simulink model "Nmpc_pathctl_casadi"  (R2022b)
(part 8 of 11)

1961.70000000000,0;1961.80000000000,0;1961.90000000000,0;1962,0;1962.10000000000,0;1962.20000000000,0;1962.30000000000,0;1962.40000000000,0;1962.50000000000,0;1962.60000000000,0;1962.70000000000,0;1962.80000000000,0;1962.90000000000,0;1963,0;1963.10000000000,0;1963.20000000000,0;1963.30000000000,0;1963.40000000000,0;1963.50000000000,0;1963.60000000000,0;1963.70000000000,0;1963.80000000000,0;1963.90000000000,0;1964,0;1964.10000000000,0;1964.20000000000,0;1964.30000000000,0;1964.40000000000,0;1964.50000000000,0;1964.60000000000,0;1964.70000000000,0;1964.80000000000,0;1964.90000000000,0;1965,0;1965.10000000000,0;1965.20000000000,0;1965.30000000000,0;1965.40000000000,0;1965.50000000000,0;1965.60000000000,0;1965.70000000000,0;1965.80000000000,0;1965.90000000000,0;1966,0;1966.10000000000,0;1966.20000000000,0;1966.30000000000,0;1966.40000000000,0;1966.50000000000,0;1966.60000000000,0;1966.70000000000,0;1966.80000000000,0;1966.90000000000,0;1967,0;1967.10000000000,0;1967.20000000000,0;1967.30000000000,0;1967.40000000000,0;1967.50000000000,0;1967.60000000000,0;1967.70000000000,0;1967.80000000000,0;1967.90000000000,0;1968,0;1968.10000000000,0;1968.20000000000,0;1968.30000000000,0;1968.40000000000,0;1968.50000000000,0;1968.60000000000,0;1968.70000000000,0;1968.80000000000,0;1968.90000000000,0;1969,0;1969.10000000000,0;1969.20000000000,0;1969.30000000000,0;1969.40000000000,0;1969.50000000000,0;1969.60000000000,0;1969.70000000000,0;1969.80000000000,0;1969.90000000000,0;1970,0;1970.10000000000,0;1970.20000000000,0;1970.30000000000,0;1970.40000000000,0;1970.50000000000,0;1970.60000000000,0;1970.70000000000,0;1970.80000000000,0;1970.90000000000,0;1971,0;1971.10000000000,0;1971.20000000000,0;1971.30000000000,0;1971.40000000000,0;1971.50000000000,0;1971.60000000000,0;1971.70000000000,0;1971.80000000000,0;1971.90000000000,0;1972,0;1972.10000000000,0;1972.20000000000,0;1972.30000000000,0;1972.40000000000,0;1972.50000000000,0;1972.60000000000,0;1972.70000000000,0;1972.80000000000,0;1972.90000000000,0;1973,0;1973.10000000000,0;1973.20000000000,0;1973.30000000000,0;1973.40000000000,0;1973.50000000000,0;1973.60000000000,0;1973.70000000000,0;1973.80000000000,0;1973.90000000000,0;1974,0;1974.10000000000,0;1974.20000000000,0;1974.30000000000,0;1974.40000000000,0;1974.50000000000,0;1974.60000000000,0;1974.70000000000,0;1974.80000000000,0;1974.90000000000,0;1975,0;1975.10000000000,0;1975.20000000000,0;1975.30000000000,0;1975.40000000000,0;1975.50000000000,0;1975.60000000000,0;1975.70000000000,0;1975.80000000000,0;1975.90000000000,0;1976,0;1976.10000000000,0;1976.20000000000,0;1976.30000000000,0;1976.40000000000,0;1976.50000000000,0;1976.60000000000,0;1976.70000000000,0;1976.80000000000,0;1976.90000000000,0;1977,0;1977.10000000000,0;1977.20000000000,0;1977.30000000000,0;1977.40000000000,0;1977.50000000000,0;1977.60000000000,0;1977.70000000000,0;1977.80000000000,0;1977.90000000000,0;1978,0;1978.10000000000,0;1978.20000000000,0;1978.30000000000,0;1978.40000000000,0;1978.50000000000,0;1978.60000000000,0;1978.70000000000,0;1978.80000000000,0;1978.90000000000,0;1979,0;1979.10000000000,0;1979.20000000000,0;1979.30000000000,0;1979.40000000000,0;1979.50000000000,0;1979.60000000000,0;1979.70000000000,0;1979.80000000000,0;1979.90000000000,0;1980,0;1980.10000000000,0;1980.20000000000,0;1980.30000000000,0;1980.40000000000,0;1980.50000000000,0;1980.60000000000,0;1980.70000000000,0;1980.80000000000,0;1980.90000000000,0;1981,0;1981.10000000000,0;1981.20000000000,0;1981.30000000000,0;1981.40000000000,0;1981.50000000000,0;1981.60000000000,0;1981.70000000000,0;1981.80000000000,0;1981.90000000000,0;1982,0;1982.10000000000,0;1982.20000000000,0;1982.30000000000,0;1982.40000000000,0;1982.50000000000,0;1982.60000000000,0;1982.70000000000,0;1982.80000000000,0;1982.90000000000,0;1983,0;1983.10000000000,0;1983.20000000000,0;1983.30000000000,0;1983.40000000000,0;1983.50000000000,0;1983.60000000000,0;1983.70000000000,0;1983.80000000000,0;1983.90000000000,0;1984,0;1984.10000000000,0;1984.20000000000,0;1984.30000000000,0;1984.40000000000,0;1984.50000000000,0;1984.60000000000,0;1984.70000000000,0;1984.80000000000,0;1984.90000000000,0;1985,0;1985.10000000000,0;1985.20000000000,0;1985.30000000000,0;1985.40000000000,0;1985.50000000000,0;1985.60000000000,0;1985.70000000000,0;1985.80000000000,0;1985.90000000000,0;1986,0;1986.10000000000,0;1986.20000000000,0;1986.30000000000,0;1986.40000000000,0;1986.50000000000,0;1986.60000000000,0;1986.70000000000,0;1986.80000000000,0;1986.90000000000,0;1987,0;1987.10000000000,0;1987.20000000000,0;1987.30000000000,0;1987.40000000000,0;1987.50000000000,0;1987.60000000000,0;1987.70000000000,0;1987.80000000000,0;1987.90000000000,0;1988,0;1988.10000000000,0;1988.20000000000,0;1988.30000000000,0;1988.40000000000,0;1988.50000000000,0;1988.60000000000,0;1988.70000000000,0;1988.80000000000,0;1988.90000000000,0;1989,0;1989.10000000000,0;1989.20000000000,0;1989.30000000000,0;1989.40000000000,0;1989.50000000000,0;1989.60000000000,0;1989.70000000000,0;1989.80000000000,0;1989.90000000000,0;1990,0;1990.10000000000,0;1990.20000000000,0;1990.30000000000,0;1990.40000000000,0;1990.50000000000,0;1990.60000000000,0;1990.70000000000,0;1990.80000000000,0;1990.90000000000,0;1991,0;1991.10000000000,0;1991.20000000000,0;1991.30000000000,0;1991.40000000000,0;1991.50000000000,0;1991.60000000000,0;1991.70000000000,0;1991.80000000000,0;1991.90000000000,0;1992,0;1992.10000000000,0;1992.20000000000,0;1992.30000000000,0;1992.40000000000,0;1992.50000000000,0;1992.60000000000,0;1992.70000000000,0;1992.80000000000,0;1992.90000000000,0;1993,0;1993.10000000000,0;1993.20000000000,0;1993.30000000000,0;1993.40000000000,0;1993.50000000000,0;1993.60000000000,0;1993.70000000000,0;1993.80000000000,0;1993.90000000000,0;1994,0;1994.10000000000,0;1994.20000000000,0;1994.30000000000,0;1994.40000000000,0;1994.50000000000,0;1994.60000000000,0;1994.70000000000,0;1994.80000000000,0;1994.90000000000,0;1995,0;1995.10000000000,0;1995.20000000000,0;1995.30000000000,0;1995.40000000000,0;1995.50000000000,0;1995.60000000000,0;1995.70000000000,0;1995.80000000000,0;1995.90000000000,0;1996,0;1996.10000000000,0;1996.20000000000,0;1996.30000000000,0;1996.40000000000,0;1996.50000000000,0;1996.60000000000,0;1996.70000000000,0;1996.80000000000,0;1996.90000000000,0;1997,0;1997.10000000000,0;1997.20000000000,0;1997.30000000000,0;1997.40000000000,0;1997.50000000000,0;1997.60000000000,0;1997.70000000000,0;1997.80000000000,0;1997.90000000000,0;1998,0;1998.10000000000,0;1998.20000000000,0;1998.30000000000,0;1998.40000000000,0;1998.50000000000,0;1998.60000000000,0;1998.70000000000,0;1998.80000000000,0;1998.90000000000,0;1999,0;1999.10000000000,0;1999.20000000000,0;1999.30000000000,0;1999.40000000000,0;1999.50000000000,0;1999.60000000000,0;1999.70000000000,0;1999.80000000000,0;1999.90000000000,0;2000,0];
            
%             plot(out.y.signals.values(:,5),out.y.signals.values(:,6))
%             hold on
%             plot(casobj.path(:,1),casobj.path(:,2))
%             plot(out.y.signals.values(:,5),out.y.signals.values(:,4))
%             plot(out.y.signals.values(:,5),out.y.signals.values(:,3))


            % 直线驾驶
